simulink model "KalmanFilter"  (R2019b)
settings: Solver=FixedStepAuto  StartTime=0.0  StopTime=10.0  FixedStep=Ts  RelTol=1e-3
values from neighbouring files (symbols this model uses):
  A = [1 1; 0 1]    [KalmanFilter_para.m]
  B = [0 1]'    [KalmanFilter_para.m]
  C = [1 0]    [KalmanFilter_para.m]
  D = 0    [KalmanFilter_para.m]
  Q = 1e-3    (= 0.001)    [KalmanFilter.m]    (also in KalmanFilter_para.m = diag([1e-3 2e-3]))
  R = 1e-3    (= 0.001)    [KalmanFilter.m]    (also in KalmanFilter_para.m = 0.1)
  Ts = 1e-3    (= 0.001)    [KalmanFilter.m]    (also in KalmanFilter_para.m)
undefined symbols (not defined in the file or in its folder): Discrete, Time
libraries: simulink x2, dsparch4 x1, ctrlSharedLib x1
settings Model: Creator=XiaoCY  LastModifiedBy=XiaoCY

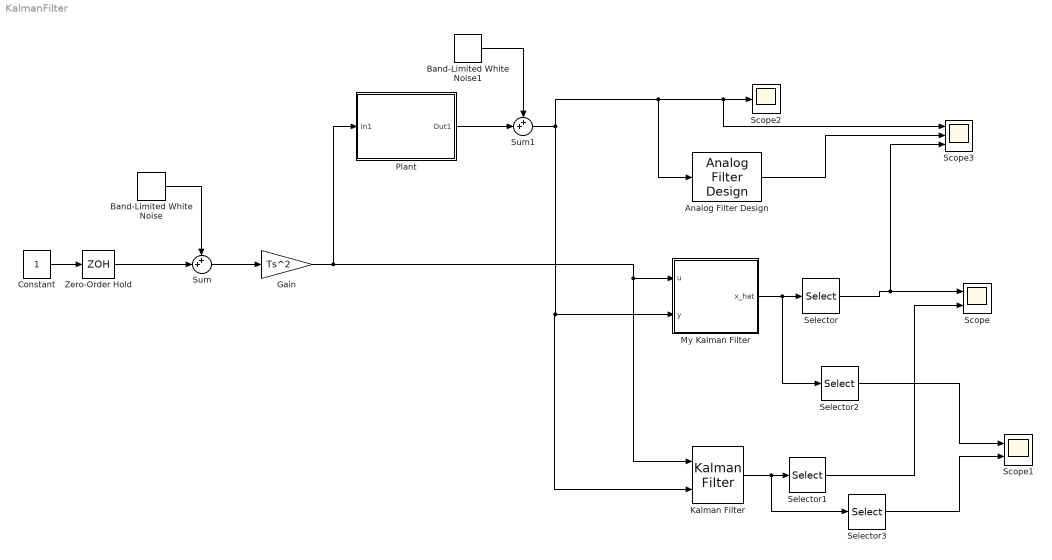
== system KalmanFilter ==
  Analog Filter Design : dsparch4/Analog Filter Design  method=Butterworth  filttype=Lowpass  N=2  Wlo=10*2*pi  Whi=80  Rp=2  Rs=40
  Band-Limited White Noise : simulink/Sources/Band-Limited White Noise  Cov=R*Ts  Ts=Ts  seed=[23341]
  Band-Limited White Noise1 : simulink/Sources/Band-Limited White Noise  Cov=R*Ts  Ts=Ts  seed=12414
  Constant : Constant
  Gain : Gain  Gain=Ts^2
  Kalman Filter : ctrlSharedLib/Kalman Filter  TimeDomain=Discrete-Time  UseCurrentEstimator=on  ModelSource=Individual A, B, C, D matrices  ModelSourceVariable=ss(0.95,1,1,0,1)  A=A  B=B  C=C  D=D  NumberOfStates=1  NumberOfInputs=1  NumberOfOutputs=1  InitialEstimateSource=Dialog  X0=0  P0=10  UseK=off  UseGH=off  NumberOfProcessNoiseInputs=1  G=1  TimeInvariantG=on  H=0  TimeInvariantH=on  Q=Q  TimeInvariantQ=on  R=R  TimeInvariantR=on  N=0  TimeInvariantN=on  AddInputPort=on  AddEnablePort=off  OutputEstimatedY=off  OutputP=off  Ts=-1
      settings: SourceProductBaseCode=CT
  My Kalman Filter : Subsystem  mask{A=A, B=B, C=C, D=D, Q=Q, R=R, Ts=Ts}
  Plant : Subsystem
  Scope : Scope  NumInputPorts=2
  Scope1 : Scope  NumInputPorts=2
  Scope2 : Scope
  Scope3 : Scope  NumInputPorts=3
  Selector : Selector  InputPortWidth=2  IndexOptions=Index vector (dialog)  Indices=1  OutputSizes=1
  Selector1 : Selector  InputPortWidth=2  IndexOptions=Index vector (dialog)  Indices=1  OutputSizes=1
  Selector2 : Selector  InputPortWidth=2  IndexOptions=Index vector (dialog)  Indices=2  OutputSizes=1
  Selector3 : Selector  InputPortWidth=2  IndexOptions=Index vector (dialog)  Indices=2  OutputSizes=1
  Sum : Sum  Inputs=++|
  Sum1 : Sum  Inputs=++|
  Zero-Order Hold : ZeroOrderHold  SampleTime=Ts
  wires:
  Constant/1 -> Zero-Order Hold/1
  My Kalman Filter/1(x_hat) -> Selector2/1, Selector/1
  Selector/1 -> Scope3/3, Scope/1
  Kalman Filter/1 -> Selector3/1, Selector1/1
  Selector1/1 -> Scope/2
  Selector2/1 -> Scope1/1
  Selector3/1 -> Scope1/2
  Gain/1 -> Kalman Filter/1, My Kalman Filter/1(u), Plant/1(In1)
  Sum/1 -> Gain/1
  Zero-Order Hold/1 -> Sum/2
  Band-Limited White Noise/1 -> Sum/1
  Band-Limited White Noise1/1 -> Sum1/1
  Sum1/1 -> Kalman Filter/2, My Kalman Filter/2(y), Analog Filter Design/1, Scope3/1, Scope2/1
  Plant/1(Out1) -> Sum1/2
  Analog Filter Design/1 -> Scope3/2

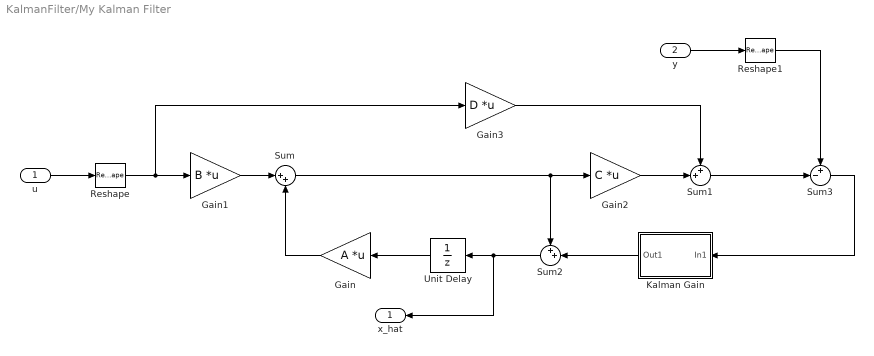
== system KalmanFilter/My Kalman Filter ==
  u : Inport
  y : Inport  Port=2
  Gain : Gain  Gain=A  Multiplication=Matrix(K*u)
  Gain1 : Gain  Gain=B  Multiplication=Matrix(K*u)
  Gain2 : Gain  Gain=C  Multiplication=Matrix(K*u)
  Gain3 : Gain  Gain=D  Multiplication=Matrix(K*u)
  Kalman Gain : Subsystem
      mask Display: disp('K')
  Reshape : Reshape  OutputDimensionality=Column vector (2-D)
  Reshape1 : Reshape  OutputDimensionality=Column vector (2-D)
  Sum : Sum  Inputs=|++
  Sum1 : Sum  Inputs=++|
  Sum2 : Sum  Inputs=++|
  Sum3 : Sum  Inputs=+-|
  Unit Delay : UnitDelay  SampleTime=-1  HasFrameUpgradeWarning=on
  x_hat : Outport
  wires:
  Unit Delay/1 -> Gain/1
  u/1 -> Reshape/1
  Gain/1 -> Sum/2
  Gain1/1 -> Sum/1
  Sum/1 -> Gain2/1, Sum2/1
  Gain2/1 -> Sum1/2
  Gain3/1 -> Sum1/1
  Sum2/1 -> x_hat/1, Unit Delay/1
  Sum1/1 -> Sum3/2
  y/1 -> Reshape1/1
  Sum3/1 -> Kalman Gain/1(In1)
  Reshape/1 -> Gain3/1, Gain1/1
  Reshape1/1 -> Sum3/1
  Kalman Gain/1(Out1) -> Sum2/2

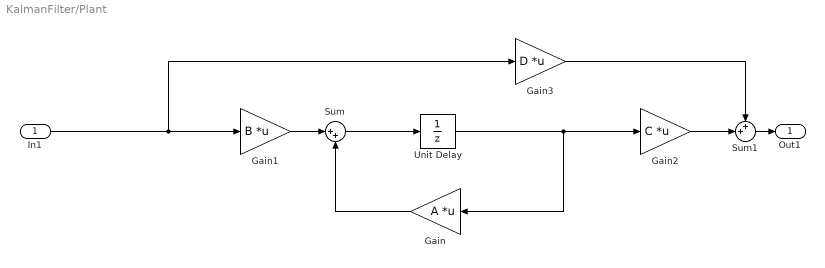
== system KalmanFilter/Plant ==
  In1 : Inport
  Gain : Gain  Gain=A  Multiplication=Matrix(K*u)
  Gain1 : Gain  Gain=B  Multiplication=Matrix(K*u)
  Gain2 : Gain  Gain=C  Multiplication=Matrix(K*u)
  Gain3 : Gain  Gain=D  Multiplication=Matrix(K*u)
  Sum : Sum  Inputs=|++
  Sum1 : Sum  Inputs=++|
  Unit Delay : UnitDelay  SampleTime=-1  HasFrameUpgradeWarning=on
  Out1 : Outport
  wires:
  Sum1/1 -> Out1/1
  In1/1 -> Gain3/1, Gain1/1
  Gain3/1 -> Sum1/1
  Gain1/1 -> Sum/1
  Gain2/1 -> Sum1/2
  Gain/1 -> Sum/2
  Unit Delay/1 -> Gain/1, Gain2/1
  Sum/1 -> Unit Delay/1

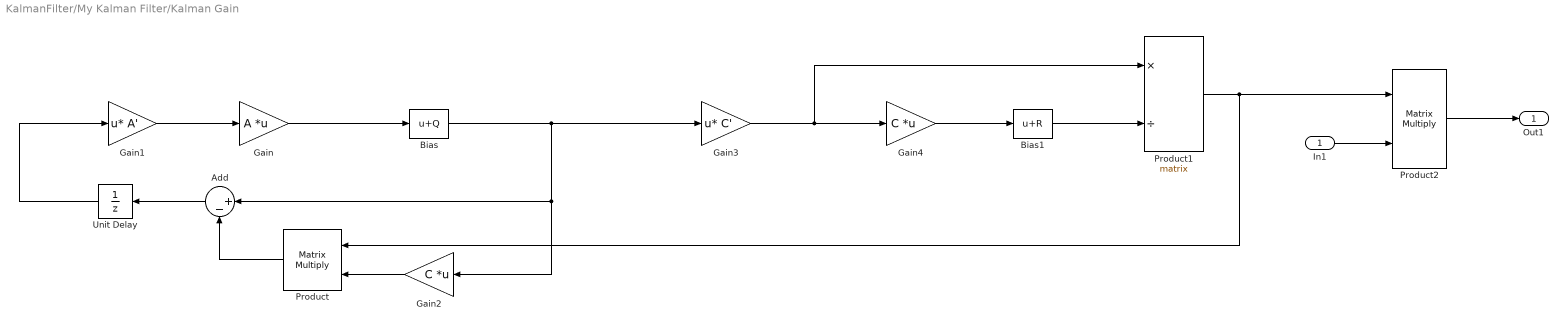
== system KalmanFilter/My Kalman Filter/Kalman Gain ==
  In1 : Inport
  Add : Sum  Inputs=|+-
  Bias : Bias  Bias=Q
  Bias1 : Bias  Bias=R
  Gain : Gain  Gain=A  Multiplication=Matrix(K*u)
  Gain1 : Gain  Gain=A'  Multiplication=Matrix(u*K)
  Gain2 : Gain  Gain=C  Multiplication=Matrix(K*u)
  Gain3 : Gain  Gain=C'  Multiplication=Matrix(u*K)
  Gain4 : Gain  Gain=C  Multiplication=Matrix(K*u)
  Product : Product  Multiplication=Matrix(*)
  Product1 : Product  Inputs=*/  Multiplication=Matrix(*)
  Product2 : Product  Multiplication=Matrix(*)
  Unit Delay : UnitDelay  SampleTime=-1  HasFrameUpgradeWarning=on
  Out1 : Outport
  wires:
  Unit Delay/1 -> Gain1/1
  Gain1/1 -> Gain/1
  Gain/1 -> Bias/1
  Bias/1 -> Gain3/1, Gain2/1, Add/1
  Gain2/1 -> Product/2
  Product/1 -> Add/2
  Add/1 -> Unit Delay/1
  Gain3/1 -> Gain4/1, Product1/1
  Gain4/1 -> Bias1/1
  Bias1/1 -> Product1/2
  Product1/1 -> Product2/1, Product/1
  In1/1 -> Product2/2
  Product2/1 -> Out1/1
